simulink model "tcpClient_InstrumentControl_UnityServer"  (R2019a)
settings: Solver=FixedStepAuto  StartTime=0.0  StopTime=30  FixedStep=0.2  RelTol=1e-3
libraries: instrumentlib x1
settings Model: Creator=FJJ  LastModifiedBy=FJJ

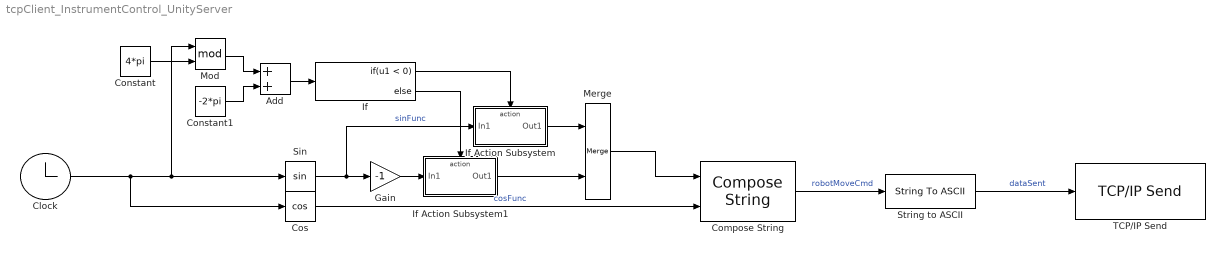
== system tcpClient_InstrumentControl_UnityServer ==
  Add : Sum
  Clock : Clock
      settings: Decimation=100
  Compose String : ComposeString  Format="\"x %.3f;z %.3f\""
  Constant : Constant  Value=4*pi
  Constant1 : Constant  Value=-2*pi
  Cos : Trigonometry  Operator=cos
  Gain : Gain  Gain=-1
  If : If  IfExpression=u1 < 0
  If Action Subsystem : Subsystem  TreatAsAtomicUnit=on
  If Action Subsystem1 : Subsystem  TreatAsAtomicUnit=on
  Merge : Merge
  Mod : Math  Operator=mod  SaturateOnIntegerOverflow=on
  Sin : Trigonometry
  String to ASCII : StringToASCII
  TCP/IP Send : instrumentlib/TCP//IP Send  Host=127.0.0.1  Port=55002  EnableBlockingMode=on  Timeout=10  ByteOrder=BigEndian  TransferDelay=on
      settings: SourceProductName=Instrument Control Toolbox
  wires:
  Cos/1 -> Compose String/2  "cosFunc"
  Clock/1 -> Mod/1, Sin/1, Cos/1
  Sin/1 -> Gain/1, If Action Subsystem/1(In1)  "sinFunc"
  Compose String/1 -> String to ASCII/1  "robotMoveCmd"
  String to ASCII/1 -> TCP/IP Send/1  "dataSent"
  Constant/1 -> Mod/2
  Mod/1 -> Add/1
  Constant1/1 -> Add/2
  Add/1 -> If/1
  If/1 -> If Action Subsystem/Action
  If/2 -> If Action Subsystem1/Action
  Gain/1 -> If Action Subsystem1/1(In1)
  If Action Subsystem/1(Out1) -> Merge/1
  If Action Subsystem1/1(Out1) -> Merge/2
  Merge/1 -> Compose String/1

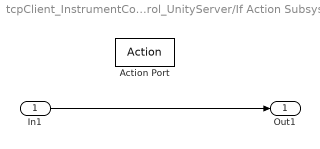
== system tcpClient_InstrumentControl_UnityServer/If Action Subsystem ==
  In1 : Inport
  Action Port : ActionPort  ActionPortLabel=if(u1 < 0)
  Out1 : Outport
  wires:
  In1/1 -> Out1/1

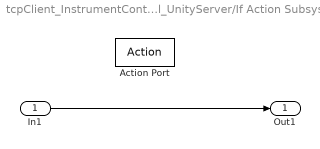
== system tcpClient_InstrumentControl_UnityServer/If Action Subsystem1 ==
  In1 : Inport
  Action Port : ActionPort  ActionPortLabel=else
  Out1 : Outport
  wires:
  In1/1 -> Out1/1
